simulink model "pumpModel"  (R2017a)
settings: Solver=VariableStepAuto  StartTime=0.0  StopTime=10.0  RelTol=1e-3
undefined symbols (not defined in the file or in its folder): k11, k12, k13, k2
settings Model: Creator=bogdan.tamas  LastModifiedBy=bogdan.tamas
settings DataIOCC: LimitDataPoints=on  SaveOutput=off  SaveTime=off
settings OptimizationCC: BlockReduction=off  BooleanDataType=off  LifeSpan=inf
settings DebuggingCC: SaveWithParameterizedLinksMsg=none  UnderspecifiedInitializationDetection=Classic  MergeDetectMultiDrivingBlocksExec=none  SignalResolutionControl=TryResolveAllWithWarning  AllowSymbolicDim=off  SFUnexpectedBacktrackingDiag=warning  SFNoUnconditionalDefaultTransitionDiag=warning  SFExecutionAtInitializationDiag=none
settings HardwareCC: TargetUnknown=on
settings GRTTargetCC: TargetLangStandard=C89/C90 (ANSI)  GeneratePreprocessorConditionals=Disable all

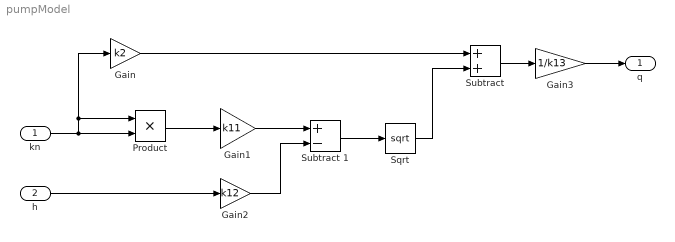
== system pumpModel ==
  kn : Inport
  h : Inport  Port=2
  Gain : Gain  Gain=k2
  Gain1 : Gain  Gain=k11
  Gain2 : Gain  Gain=k12
  Gain3 : Gain  Gain=1/k13
  Product : Product
  Sqrt : Sqrt  SaturateOnIntegerOverflow=on
  "Subtract " : Sum
  Subtract 1 : Sum  Inputs=+-
  q : Outport
  wires:
  h/1 -> Gain2/1
  kn/1 -> Product/2, Product/1, Gain/1
  Gain/1 -> "Subtract "/1
  Sqrt/1 -> "Subtract "/2
  "Subtract "/1 -> Gain3/1
  Gain3/1 -> q/1
  Product/1 -> Gain1/1
  Gain2/1 -> Subtract 1/2
  Gain1/1 -> Subtract 1/1
  Subtract 1/1 -> Sqrt/1
